simulink model "soh_sfun"  (R2015b)
settings: Solver=FixedStepDiscrete  StartTime=0.0  StopTime=inf  RelTol=1e-3
values from neighbouring files (symbols this model uses):
  sohv_factoryInit_sohc = ones(40,1)    [SOH_ini.m]
undefined symbols (not defined in the file): bmsc_InternalDischgResistX, bmsc_InternalDischgResistY, bmsc_InternalDischgResistZ, sohc_current_threshold, sohc_customer_filter_coeff, sohc_filter_coeff, sohc_pct_R_limit, sohk_CellBalancingResistor, sohv_factoryInit_sohr
settings Model: TunableVars=bmsc_InternalChgResistX,bmsc_InternalChgResistY,bmsc_InternalChgResistZ,bmsc_InternalDischgResistX,bmsc_InternalDischgResistY,bmsc_InternalDischgResistZ,sohc_current_threshold,sohc_customer_filter_coeff,sohc_filter_coeff,sohc_pct_R_limit,sohk_CellBalancingResistor,sohk_delta_time,sohk_stepSize,sohv_factoryInit_sohc,sohv_factoryInit_sohr  TunableVarsStorageClass=Auto,Auto,Auto,Auto,Auto,Auto,Auto,Auto,Auto,Auto,Auto,Auto,Auto,Auto,Auto  TunableVarsTypeQualifier=,,,,,,,,,,,,,,  Creator=nctzv8  LastModifiedBy=nctzv8
settings ConfigSet: Description=OpenECU configuration set for code generation under RTW-EC.
settings SolverCC: PositivePriorityOrder=on
settings DataIOCC: SaveFormat=Array  SignalLoggingSaveFormat=ModelDataLogs
settings OptimizationCC: DefaultParameterBehavior=Inlined  InlineInvariantSignals=on  ExpressionDepthLimit=2147483647  StateBitsets=on  DataBitsets=on  ZeroExternalMemoryAtStartup=off  ZeroInternalMemoryAtStartup=off  NoFixptDivByZeroProtection=on  EfficientFloat2IntCast=on  OptimizeModelRefInitCode=on  LifeSpan=1
settings DebuggingCC: SaveWithParameterizedLinksMsg=none  UnderspecifiedInitializationDetection=Classic  MergeDetectMultiDrivingBlocksExec=none  SignalResolutionControl=TryResolveAllWithWarning  MultiTaskDSMMsg=warning  MultiTaskCondExecSysMsg=none  SingleTaskRateTransMsg=error  CheckMatrixSingularityMsg=warning  VectorMatrixConversionMsg=warning  FcnCallInpInsideContextMsg=UseLocalSettings  SignalLabelMismatchMsg=warning  StateNameClashWarn=warning
settings HardwareCC: ProdBitPerPointer=32  ProdLargestAtomicInteger=Long  ProdLargestAtomicFloat=Double  ProdEndianess=BigEndian  ProdWordSize=32  ProdHWDeviceType=Freescale->32-bit PowerPC  TargetIntDivRoundTo=Zero  TargetEndianess=BigEndian  TargetHWDeviceType=Freescale->32-bit PowerPC  ProdEqTarget=off
settings RTWCC: SystemTargetFile=openecu_ert.tlc  MakeCommand=make_rtw optimized_floating_point=1  TemplateMakefile=openecu_ert_r2015b_64.tmf  Description=OpenECU Platform Target (ERT, optimised floating-point code)  RetainRTWFile=on  IncludeHyperlinkInReport=on
settings CodeAppCC: ForceParamTrailComments=on  IgnoreCustomStorageClasses=off  SimulinkDataObjDesc=on  CustomSymbolStrType=$N$R$M  InsertBlockDesc=on  InternalIdentifier=Classic
settings STFCustomTargetCC: TargetLibSuffix=.a  GenerateSampleERTMain=on  ConcurrentExecutionCompliant=off  IncludeMdlTerminateFcn=off  GeneratePreprocessorConditionals=Use local settings  CombineOutputUpdateFcns=on  IncludeFileDelimiter=UseQuote  ERTCustomFileBanners=on  SupportContinuousTime=off  MATLABClassNameForMDSCustomization=Simulink.SoftwareTarget.ERTCustomization  CPPClassGenCompliant=off  GRTInterface=off  SystemTargetFile=openecu_ert.tlc
settings ERTTargetCC: GenerateSampleERTMain=on  ParMdlRefBuildCompliant=off  CompOptLevelCompliant=off  ConcurrentExecutionCompliant=off  IncludeMdlTerminateFcn=off  ERTFirstTimeCompliant=off  IncludeFileDelimiter=UseQuote  SupportNonInlinedSFcns=on  ModelStepFunctionPrototypeControlCompliant=off  CPPClassGenCompliant=off  UseToolchainInfoCompliant=off  ExtModeMexFile=noextcomm  InlinedParameterPlacement=NonHierarchical  ERTSrcFileBannerTemplate=oe_code_c_template.cgt  ERTHdrFileBannerTemplate=oe_code_h_template.cgt  ERTDataSrcFileTemplate=oe_data_c_template.cgt  ERTDataHdrFileTemplate=oe_data_h_template.cgt  ERTCustomFileTemplate=example_file_process.tlc  GlobalDataDefinition=InSeparateSourceFile  GlobalDataReference=InSeparateHeaderFile  EnableUserReplacementTypes=on

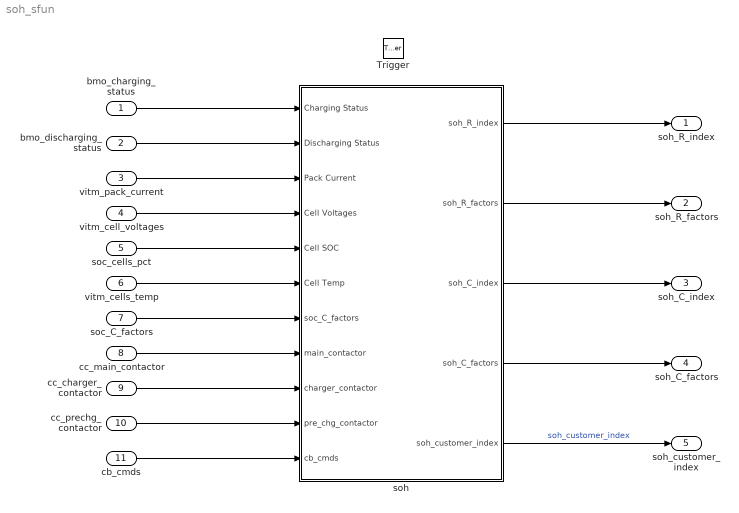
== system soh_sfun ==
  bmo_charging_status : Inport
  bmo_discharging_status : Inport  Port=2
  vitm_pack_current : Inport  Port=3
  vitm_cell_voltages : Inport  Port=4  PortDimensions=40
  soc_cells_pct : Inport  Port=5  PortDimensions=40
  vitm_cells_temp : Inport  Port=6  PortDimensions=40
  soc_C_factors : Inport  Port=7  PortDimensions=40
  cc_main_contactor : Inport  Port=8
  cc_charger_contactor : Inport  Port=9
  cc_prechg_contactor : Inport  Port=10
  cb_cmds : Inport  Port=11  OutDataTypeStr=boolean  PortDimensions=40
  Trigger : TriggerPort  TriggerType=function-call  PortDimensions=1
  soh : Subsystem  mask{sfcnParam1=bmsc_InternalDischgResistX, sfcnParam2=bmsc_InternalDischgResistY, sfcnParam3=bmsc_InternalDischgResistZ, sfcnParam4=sohc_current_threshold, sfcnParam5=sohc_customer_filter_coeff, sfcnParam6=sohc_filter_coeff, sfcnParam7=sohc_pct_R_limit, sfcnParam8=sohk_CellBalancingResistor, sfcnParam9=sohv_factoryInit_sohc, sfcnParam10=sohv_factoryInit_sohr}
      mask prompts: sfcnParam1 "bmsc_InternalDischgResistX:"; sfcnParam2 "bmsc_InternalDischgResistY:"; sfcnParam3 "bmsc_InternalDischgResistZ:"; sfcnParam4 "sohc_current_threshold:"; sfcnParam5 "sohc_customer_filter_coeff:"; sfcnParam6 "sohc_filter_coeff:"; sfcnParam7 "sohc_pct_R_limit:"; sfcnParam8 "sohk_CellBalancingResistor:"; sfcnParam9 "sohv_factoryInit_sohc:"; sfcnParam10 "sohv_factoryInit_sohr:"
      mask help: Simulink:masks:GenSFuncDesc_MD
      mask Help: eval('feval(''rtwprivate'',''rtwhelpview'',''rtw_sfcn_block'')');
  soh_R_index : Outport
  soh_R_factors : Outport  Port=2  PortDimensions=40
  soh_C_index : Outport  Port=3
  soh_C_factors : Outport  Port=4  PortDimensions=40  InitialOutput=sohv_factoryInit_sohc
  soh_customer_index : Outport  Port=5
  wires:
  bmo_charging_status/1 -> soh/1(Charging Status)
  bmo_discharging_status/1 -> soh/2(Discharging Status)
  vitm_pack_current/1 -> soh/3(Pack Current)
  vitm_cell_voltages/1 -> soh/4(Cell Voltages)
  soc_cells_pct/1 -> soh/5(Cell SOC)
  vitm_cells_temp/1 -> soh/6(Cell Temp)
  soc_C_factors/1 -> soh/7(soc_C_factors)
  cc_main_contactor/1 -> soh/8(main_contactor)
  cc_charger_contactor/1 -> soh/9(charger_contactor)
  cc_prechg_contactor/1 -> soh/10(pre_chg_contactor)
  cb_cmds/1 -> soh/11(cb_cmds)
  soh/1(soh_R_index) -> soh_R_index/1
  soh/4(soh_C_factors) -> soh_C_factors/1
  soh/3(soh_C_index) -> soh_C_index/1
  soh/2(soh_R_factors) -> soh_R_factors/1
  soh/5(soh_customer_index) -> soh_customer_index/1  "soh_customer_index"

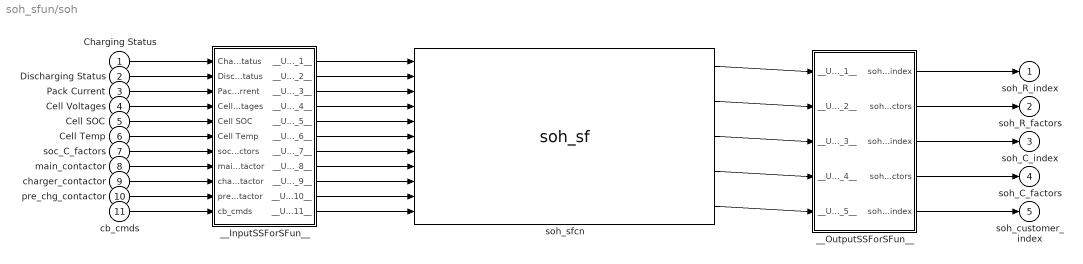
== system soh_sfun/soh ==
  Charging Status : Inport  OutDataTypeStr=boolean
  Discharging Status : Inport  Port=2  OutDataTypeStr=boolean
  Pack Current : Inport  Port=3
  Cell Voltages : Inport  Port=4  PortDimensions=40
  Cell SOC : Inport  Port=5  PortDimensions=40
  Cell Temp : Inport  Port=6  PortDimensions=40
  soc_C_factors : Inport  Port=7  PortDimensions=40
  main_contactor : Inport  Port=8
  charger_contactor : Inport  Port=9
  pre_chg_contactor : Inport  Port=10
  cb_cmds : Inport  Port=11  PortDimensions=40
  __InputSSForSFun__ : Subsystem
  __OutputSSForSFun__ : Subsystem
  soh_sfcn : S-Function  FunctionName=soh_sf  Parameters=sfcnParam1, sfcnParam2, sfcnParam3, sfcnParam4, sfcnParam5, sfcnParam6, sfcnParam7, sfcnParam8, sfcnParam9, sfcnParam10  SFunctionModules=""  SFunctionDeploymentMode=off  EnableBusSupport=off  mask{rtw_sf_name=soh_sf, showVar=off, sfcnParam1=sfcnParam1, sfcnParam2=sfcnParam2, sfcnParam3=sfcnParam3, sfcnParam4=sfcnParam4, sfcnParam5=sfcnParam5, sfcnParam6=sfcnParam6, sfcnParam7=sfcnParam7, sfcnParam8=sfcnParam8, sfcnParam9=sfcnParam9, sfcnParam10=sfcnParam10}
      mask prompts: rtw_sf_name "Simulink:masks:GenSFuncName_MP"; showVar "Simulink:masks:GenSFuncShowModuleList_MP"; sfcnParam1 "bmsc_InternalDischgResistX:"; sfcnParam2 "bmsc_InternalDischgResistY:"; sfcnParam3 "bmsc_InternalDischgResistZ:"; sfcnParam4 "sohc_current_threshold:"; sfcnParam5 "sohc_customer_filter_coeff:"; sfcnParam6 "sohc_filter_coeff:"; sfcnParam7 "sohc_pct_R_limit:"; sfcnParam8 "sohk_CellBalancingResistor:"; sfcnParam9 "sohv_factoryInit_sohc:"; sfcnParam10 "sohv_factoryInit_sohr:"
      mask help: Simulink:masks:GenSFuncDesc_MD
      mask init:
      | displist = '';
      | if ~strcmp(get_param(gcb, 'FunctionName'), rtw_sf_name);
      |   set_param(gcb, 'FunctionName', rtw_sf_name);
      | end
      | % Check if we are generating code
      | rtw_mode = false;
      | if strcmpi(get_param(bdroot(gcb),'SimulationStatus'),'Initializing')
      | 	rtw_mode = strcmpi(get_param(bdroot(gcb),'BuildingRTWCode'),'on') && ...
      | 		~strcmpi(get_param(bdroot(gcb),'TargetStyle'),'SimulationTarget');
      | end
      | if showVar || rtw_mode
      | 	if exist('rtwsfunc') == 2 | exist('rtwsfunc') == 6
      | 		tmplist = rtwsfunc(rtw_sf_name,gcb);
      | 		tmplist = DAStudio.message('Simulink:masks:GenSFuncListOfModules_IC', tmplist);
      | 	elseif showVar
      | 		tmplist1 = DAStudio.message('Simulink:masks:GenSFuncListOfModules_IC', '');
      |         tmplist2 = DAStudio.message('Simulink:masks:GenSFuncNotLicensed_IC');
      |         tmplist = [tmplist1 tmplist2];
      |  	end
      | end
      | if showVar
      |   displist = tmplist;
      | end
      settings: CopyFcn=|
      | if ~strcmp(get_param(gcb,'Linkstatus'),'none') && ...
      | ~strcmp(get_param(gcb,'Linkstatus'),'implicit')
      |   set_param(gcb,'LinkStatus','none');
      | end
      mask Help: eval('feval(''rtwprivate'',''rtwhelpview'',''rtw_sfcn_block'')');
      mask Display:
      | port_label('input',1,'Charging Status');
      | port_label('input',2,'Discharging Status');
      | port_label('input',3,'Pack Current');
      | port_label('input',4,'Cell Voltages');
      | port_label('input',5,'Cell SOC');
      | port_label('input',6,'Cell Temp');
      | port_label('input',7,'soc_C_factors');
      | port_label('input',8,'main_contactor');
      | port_label('input',9,'charger_contactor');
      | port_label('input',10,'pre_chg_contactor');
      | port_label('input',11,'cb_cmds');
      | port_label('output',1,'soh_R_index');
      | port_label('output',2,'soh_R_factors');
      | port_label('output',3,'soh_C_index');
      | port_label('output',4,'soh_C_factors');
      | port_label('output',5,'soh_customer_index');
  soh_R_index : Outport
  soh_R_factors : Outport  Port=2
  soh_C_index : Outport  Port=3
  soh_C_factors : Outport  Port=4  PortDimensions=40
  soh_customer_index : Outport  Port=5
  wires:
  Charging Status/1 -> __InputSSForSFun__/1(Charging Status)
  Discharging Status/1 -> __InputSSForSFun__/2(Discharging Status)
  Pack Current/1 -> __InputSSForSFun__/3(Pack Current)
  Cell Voltages/1 -> __InputSSForSFun__/4(Cell Voltages)
  Cell SOC/1 -> __InputSSForSFun__/5(Cell SOC)
  Cell Temp/1 -> __InputSSForSFun__/6(Cell Temp)
  soc_C_factors/1 -> __InputSSForSFun__/7(soc_C_factors)
  main_contactor/1 -> __InputSSForSFun__/8(main_contactor)
  charger_contactor/1 -> __InputSSForSFun__/9(charger_contactor)
  pre_chg_contactor/1 -> __InputSSForSFun__/10(pre_chg_contactor)
  cb_cmds/1 -> __InputSSForSFun__/11(cb_cmds)
  __InputSSForSFun__/1(__UniqueOutportName__1__) -> soh_sfcn/1
  __InputSSForSFun__/2(__UniqueOutportName__2__) -> soh_sfcn/2
  __InputSSForSFun__/3(__UniqueOutportName__3__) -> soh_sfcn/3
  __InputSSForSFun__/4(__UniqueOutportName__4__) -> soh_sfcn/4
  __InputSSForSFun__/5(__UniqueOutportName__5__) -> soh_sfcn/5
  __InputSSForSFun__/6(__UniqueOutportName__6__) -> soh_sfcn/6
  __InputSSForSFun__/7(__UniqueOutportName__7__) -> soh_sfcn/7
  __InputSSForSFun__/8(__UniqueOutportName__8__) -> soh_sfcn/8
  __InputSSForSFun__/9(__UniqueOutportName__9__) -> soh_sfcn/9
  __InputSSForSFun__/10(__UniqueOutportName__10__) -> soh_sfcn/10
  __InputSSForSFun__/11(__UniqueOutportName__11__) -> soh_sfcn/11
  soh_sfcn/1 -> __OutputSSForSFun__/1(__UniqueInportName__1__)
  soh_sfcn/2 -> __OutputSSForSFun__/2(__UniqueInportName__2__)
  soh_sfcn/3 -> __OutputSSForSFun__/3(__UniqueInportName__3__)
  soh_sfcn/4 -> __OutputSSForSFun__/4(__UniqueInportName__4__)
  soh_sfcn/5 -> __OutputSSForSFun__/5(__UniqueInportName__5__)
  __OutputSSForSFun__/1(soh_R_index) -> soh_R_index/1
  __OutputSSForSFun__/2(soh_R_factors) -> soh_R_factors/1
  __OutputSSForSFun__/3(soh_C_index) -> soh_C_index/1
  __OutputSSForSFun__/4(soh_C_factors) -> soh_C_factors/1
  __OutputSSForSFun__/5(soh_customer_index) -> soh_customer_index/1

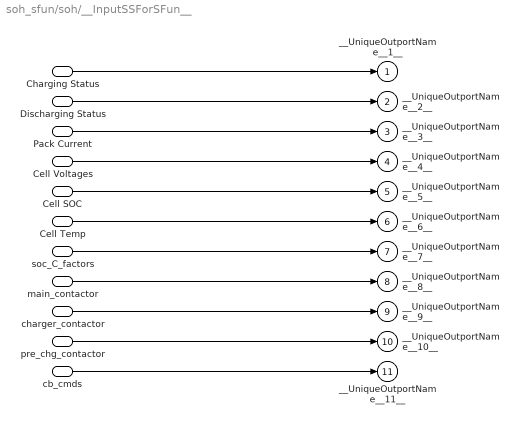
== system soh_sfun/soh/__InputSSForSFun__ ==
  Charging Status : Inport  OutDataTypeStr=boolean
  Discharging Status : Inport  Port=2  OutDataTypeStr=boolean
  Pack Current : Inport  Port=3
  Cell Voltages : Inport  Port=4  PortDimensions=40
  Cell SOC : Inport  Port=5  PortDimensions=40
  Cell Temp : Inport  Port=6  PortDimensions=40
  soc_C_factors : Inport  Port=7  PortDimensions=40
  main_contactor : Inport  Port=8
  charger_contactor : Inport  Port=9
  pre_chg_contactor : Inport  Port=10
  cb_cmds : Inport  Port=11  PortDimensions=40
  __UniqueOutportName__1__ : Outport
  __UniqueOutportName__2__ : Outport  Port=2
  __UniqueOutportName__3__ : Outport  Port=3
  __UniqueOutportName__4__ : Outport  Port=4
  __UniqueOutportName__5__ : Outport  Port=5
  __UniqueOutportName__6__ : Outport  Port=6
  __UniqueOutportName__7__ : Outport  Port=7
  __UniqueOutportName__8__ : Outport  Port=8
  __UniqueOutportName__9__ : Outport  Port=9
  __UniqueOutportName__10__ : Outport  Port=10
  __UniqueOutportName__11__ : Outport  Port=11
  wires:
  Charging Status/1 -> __UniqueOutportName__1__/1
  Discharging Status/1 -> __UniqueOutportName__2__/1
  Pack Current/1 -> __UniqueOutportName__3__/1
  Cell Voltages/1 -> __UniqueOutportName__4__/1
  Cell SOC/1 -> __UniqueOutportName__5__/1
  Cell Temp/1 -> __UniqueOutportName__6__/1
  soc_C_factors/1 -> __UniqueOutportName__7__/1
  main_contactor/1 -> __UniqueOutportName__8__/1
  charger_contactor/1 -> __UniqueOutportName__9__/1
  pre_chg_contactor/1 -> __UniqueOutportName__10__/1
  cb_cmds/1 -> __UniqueOutportName__11__/1

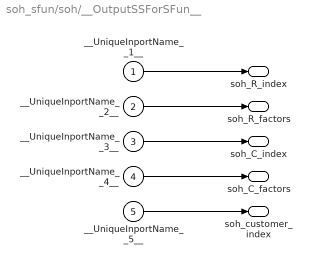
== system soh_sfun/soh/__OutputSSForSFun__ ==
  __UniqueInportName__1__ : Inport
  __UniqueInportName__2__ : Inport  Port=2
  __UniqueInportName__3__ : Inport  Port=3
  __UniqueInportName__4__ : Inport  Port=4
  __UniqueInportName__5__ : Inport  Port=5
  soh_R_index : Outport
  soh_R_factors : Outport  Port=2
  soh_C_index : Outport  Port=3
  soh_C_factors : Outport  Port=4  PortDimensions=40
  soh_customer_index : Outport  Port=5
  wires:
  __UniqueInportName__1__/1 -> soh_R_index/1
  __UniqueInportName__2__/1 -> soh_R_factors/1
  __UniqueInportName__3__/1 -> soh_C_index/1
  __UniqueInportName__4__/1 -> soh_C_factors/1
  __UniqueInportName__5__/1 -> soh_customer_index/1
